simulink model "ex2"  (Simulink 6.3)
settings: Solver=ode45  StartTime=0.0  StopTime=10.0  MaxStep=0.001  RelTol=1e-3
undefined symbols (not defined in the file or in its folder): Fs, get, magnitude
libraries: dspsnks4 x2, commanapbnd2 x1, dspstat3 x1, commrandsrc2 x1
settings Model: LastModifiedBy=lxy

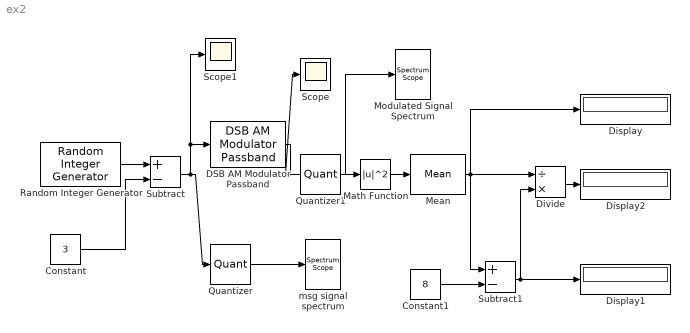
== system ex2 ==
  Constant : Constant  Value=3
  Constant1 : Constant  Value=8
  DSB AM Modulator Passband : commanapbnd2/DSB AM Modulator Passband  Fc=100  Ph=0  Offset=4
  Display : Display
  Display1 : Display
  Display2 : Display
  Divide : Product  Inputs=/*  OutScaling=2^-10
  Math Function : Math  Operator=magnitude^2  SaturateOnIntegerOverflow=on
  Mean : dspstat3/Mean  DialogController=dspDDGCreate  DialogControllerArgs=DataTag0  run=on  reset_popup=None  roundingMode=Floor  overflowMode=off
  "Modulated Signal Spectrum " : dspsnks4/Spectrum Scope  DialogController=dspdialog.SpectrumScope  DialogControllerArgs=DataTag1  ScopeProperties=on  Domain=Frequency  HorizSpan=1  UseBuffer=on  BufferSize=512  Overlap=256  inpFftLenInherit=on  FFTlength=512  numAvg=2  DisplayProperties=off  AxisGrid=on  Memory=off  FrameNumber=on  AxisLegend=off  AxisZoom=off  OpenScopeAtSimStart=on  OpenScopeImmediately=off  FigPos=get(0,'defaultfigureposition')  AxisProperties=off  XUnits=Hertz  XRange=[-Fs/2...Fs/2]  InheritXIncr=on  XIncr=1.0  XLabel=Samples  YUnits=dB  YLabel=Magnitude, dB  LineProperties=off  wintypeSpecScope=Hann  RsSpecScope=50  betaSpecScope=5  winsampSpecScope=Periodic
      settings: YMin=-50  YMax=50
  Quantizer : Quantizer  QuantizationInterval=0.001  LinearizeAsGain=off  SampleTime=0.001
  Quantizer1 : Quantizer  QuantizationInterval=0.001  LinearizeAsGain=off  SampleTime=0.001
  Random Integer Generator : commrandsrc2/Random Integer Generator  mul=7  seed=1234  Ts=1/10  frameBased=off  sampPerFrame=10  orient=off  outDataType=double
  Scope : Scope
      settings: YMin=-20  YMax=20
  Scope1 : Scope
      settings: YMin=-20  YMax=20
  Subtract : Sum  Inputs=+-  OutScaling=2^-10
  Subtract1 : Sum  Inputs=+-  OutScaling=2^-10
  msg signal spectrum : dspsnks4/Spectrum Scope  DialogController=dspdialog.SpectrumScope  DialogControllerArgs=DataTag2  ScopeProperties=on  Domain=Frequency  HorizSpan=1  UseBuffer=on  BufferSize=512  Overlap=256  inpFftLenInherit=on  FFTlength=512  numAvg=2  DisplayProperties=off  AxisGrid=on  Memory=off  FrameNumber=on  AxisLegend=off  AxisZoom=off  OpenScopeAtSimStart=on  OpenScopeImmediately=off  FigPos=get(0,'defaultfigureposition')  AxisProperties=off  XUnits=Hertz  XRange=[-Fs/2...Fs/2]  InheritXIncr=on  XIncr=1.0  XLabel=Samples  YUnits=dB  YLabel=Magnitude, dB  LineProperties=off  wintypeSpecScope=Hann  RsSpecScope=50  betaSpecScope=5  winsampSpecScope=Periodic
      settings: YMin=-50  YMax=50
  wires:
  DSB AM Modulator Passband/1 -> Quantizer1/1, Scope/1
  Quantizer1/1 -> "Modulated Signal Spectrum "/1, Math Function/1
  Random Integer Generator/1 -> Subtract/1
  Constant/1 -> Subtract/2
  Quantizer/1 -> msg signal spectrum/1
  Mean/1 -> Subtract1/1, Display/1, Divide/1
  Constant1/1 -> Subtract1/2
  Divide/1 -> Display2/1
  Math Function/1 -> Mean/1
  Subtract1/1 -> Display1/1, Divide/2
  Subtract/1 -> DSB AM Modulator Passband/1, Scope1/1, Quantizer/1
